simulink model "Cruise_Control_Simulink"  (R2018a)
settings: Solver=FixedStepAuto  StartTime=0.0  StopTime=30  FixedStep=0.01  RelTol=1e-3
values from neighbouring files (symbols this model uses):
  b = 25    [Cruise_Control_Simulink_Data.mat]
  Kd = 50    [Cruise_Control_Simulink_Data.mat]
  Ki = 15    [Cruise_Control_Simulink_Data.mat]
  Kp = 150    [Cruise_Control_Simulink_Data.mat]
  m = 1000    [Cruise_Control_Simulink_Data.mat]    (also in Lateral_Vehicle_Dynamics_Error_Model_Parameters.m = 1573)
settings Model: Creator=op95w  LastModifiedBy=op95w

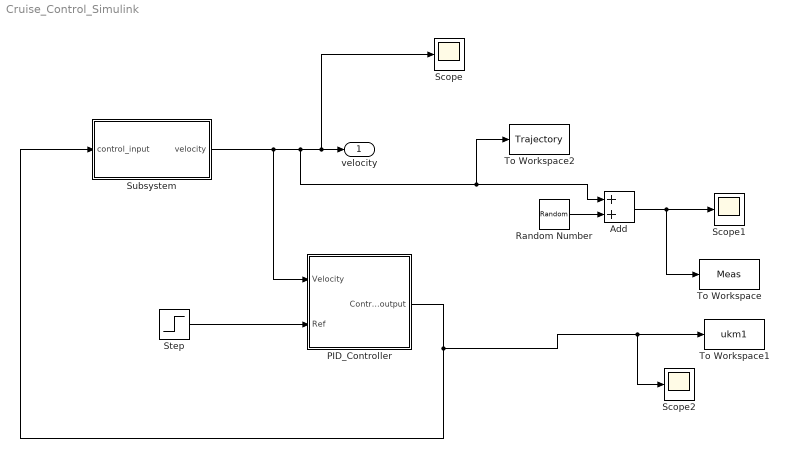
== system Cruise_Control_Simulink ==
  Add : Sum
  PID_Controller : Subsystem
  Random Number : RandomNumber  Variance=0.1
  Scope : Scope
  Scope1 : Scope
  Scope2 : Scope
  Step : Step  Time=100  Before=1  After=3  SampleTime=0
  Subsystem : Subsystem
  To Workspace : ToWorkspace  VariableName=Meas  SaveFormat=Timeseries  SampleTime=-1
  To Workspace1 : ToWorkspace  VariableName=ukm1  SaveFormat=Timeseries  SampleTime=-1
  To Workspace2 : ToWorkspace  VariableName=Trajectory  SaveFormat=Timeseries  SampleTime=-1
  velocity : Outport
  wires:
  Subsystem/1(velocity) -> PID_Controller/1(Velocity), To Workspace2/1, Add/1, Scope/1, velocity/1
  Step/1 -> PID_Controller/2(Ref)
  PID_Controller/1(Control_output) -> Scope2/1, To Workspace1/1, Subsystem/1("control_input ")
  Random Number/1 -> Add/2
  Add/1 -> To Workspace/1, Scope1/1

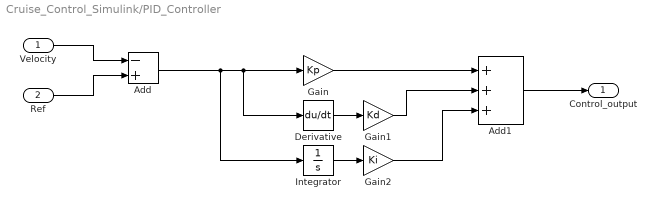
== system Cruise_Control_Simulink/PID_Controller ==
  Velocity : Inport
  Ref : Inport  Port=2
  Add : Sum  Inputs=-+
  Add1 : Sum  Inputs=3
  Derivative : Derivative
  Gain : Gain  Gain=Kp
  Gain1 : Gain  Gain=Kd
  Gain2 : Gain  Gain=Ki
  Integrator : Integrator
  Control_output : Outport
  wires:
  Ref/1 -> Add/2
  Velocity/1 -> Add/1
  Add1/1 -> Control_output/1
  Integrator/1 -> Gain2/1
  Derivative/1 -> Gain1/1
  Add/1 -> Integrator/1, Derivative/1, Gain/1
  Gain/1 -> Add1/1
  Gain1/1 -> Add1/2
  Gain2/1 -> Add1/3

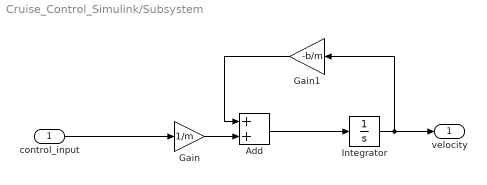
== system Cruise_Control_Simulink/Subsystem ==
  "control_input " : Inport
  Add : Sum
  Gain : Gain  Gain=1/m
  Gain1 : Gain  Gain=-b/m
  Integrator : Integrator  InitialCondition=5
  velocity : Outport
  wires:
  Integrator/1 -> velocity/1, Gain1/1
  Add/1 -> Integrator/1
  Gain/1 -> Add/2
  "control_input "/1 -> Gain/1
  Gain1/1 -> Add/1
